simulink model "SystemModelLQR"  (R2015a)
settings: Solver=ode45  StartTime=0.0  StopTime=T  RelTol=1e-3
values from neighbouring files (symbols this model uses):
  A = [3.92291500745 1 0 0 -5.78414696994 0 1 0 3.79889038796 0 0 1 ... (16 elements, 4x4)]    [ssfinal.mat]
  B = [1 0 0 0]    [ssfinal.mat]
  C = [0 0.000180250108713 -0.000200069339657 0]    [ssfinal.mat]
  fs = 100    [codigo_pt2_grupo51.m]
undefined symbols (not defined in the file or in its folder): K
settings Model: Creator=Diogo  LastModifiedBy=User

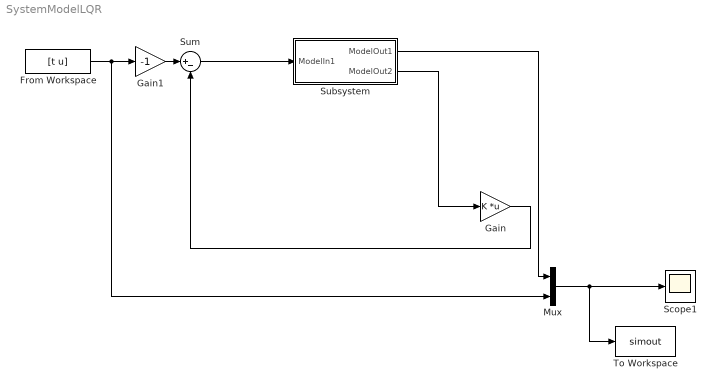
== system SystemModelLQR ==
  From Workspace : FromWorkspace  VariableName=[t u]  SampleTime=1/fs
  Gain : Gain  Gain=K  Multiplication=Matrix(K*u)
  Gain1 : Gain  Gain=-1
  Mux : Mux  Inputs=2
  Scope1 : Scope
  Subsystem : Subsystem
  Sum : Sum  Inputs=|+-
  To Workspace : ToWorkspace  VariableName=simout  SaveFormat=Structure With Time  SampleTime=-1
  wires:
  Sum/1 -> Subsystem/1(ModelIn1)
  Subsystem/2(ModelOut2) -> Gain/1
  From Workspace/1 -> Mux/2, Gain1/1
  Mux/1 -> To Workspace/1, Scope1/1
  Subsystem/1(ModelOut1) -> Mux/1
  Gain/1 -> Sum/2
  Gain1/1 -> Sum/1

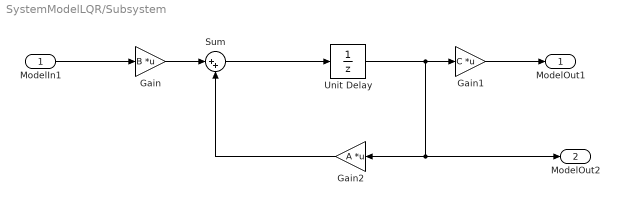
== system SystemModelLQR/Subsystem ==
  ModelIn1 : Inport
  Gain : Gain  Gain=B  Multiplication=Matrix(K*u)
  Gain1 : Gain  Gain=C  Multiplication=Matrix(K*u)
  Gain2 : Gain  Gain=A  Multiplication=Matrix(K*u)
  Sum : Sum  Inputs=|++
  Unit Delay : UnitDelay  SampleTime=-1
  ModelOut1 : Outport
  ModelOut2 : Outport  Port=2
  wires:
  Gain/1 -> Sum/1
  Sum/1 -> Unit Delay/1
  Unit Delay/1 -> Gain2/1, ModelOut2/1, Gain1/1
  Gain2/1 -> Sum/2
  ModelIn1/1 -> Gain/1
  Gain1/1 -> ModelOut1/1
